simulink model "stabilization"  (R2022b)
settings: Solver=ode14x  StartTime=0.0  StopTime=100  RelTol=1e-3  EnableMultiTasking=on
InitFcn:
  | load regulator.mat
  | load rand_stabilisation.mat
values from neighbouring files (symbols this model uses):
  P = [1 -2 2; -1 2 -1; 1 1 0]    [rand_stabilisation.m]
  Q = transpose([0 0 1])    [rand_stabilisation.m]
undefined symbols (not defined in the file or in its folder): C
settings Model: Creator=torre  LastModifiedBy=anver
settings SolverCC: AlgebraicLoopSolver=TrustRegion  AutoInsertRateTranBlk=on
settings DataIOCC: SaveOutput=off  SaveTime=off
settings OptimizationCC: DefaultParameterBehavior=Inlined  InlineInvariantSignals=on  EnhancedBackFolding=on  PassReuseOutputArgsAs=Individual arguments  StateBitsets=on  DataBitsets=on  ZeroExternalMemoryAtStartup=off  ZeroInternalMemoryAtStartup=off  NoFixptDivByZeroProtection=on  LifeSpan=1  OptimizeBlockOrder=speed  DifferentSizesBufferReuse=on  EfficientTunableParamExpr=on
settings DebuggingCC: ParameterTunabilityLossMsg=error  UnconnectedInputMsg=warning  UnconnectedOutputMsg=warning  UnconnectedLineMsg=warning
settings HardwareCC: ProdBitPerPointer=32  ProdBitPerSizeT=32  ProdBitPerPtrDiffT=32  ProdLargestAtomicFloat=None  ProdIntDivRoundTo=Floor  ProdWordSize=32  ProdHWDeviceType=Generic->Custom
settings ModelReferenceCC: EnableRefExpFcnMdlSchedulingChecks=on
settings SFSimCC: MATLABDynamicMemAlloc=off
settings RTWCC: Description=Embedded Coder  SystemTargetFile=ert.tlc  TLCOptions=-p0  GenCodeOnly=on  TemplateMakefile=ert_default_tmf  GenerateReport=on  RTWVerbose=off  IncludeHyperlinkInReport=on  LaunchReport=on  DLArmComputeVersion=19.05
settings CodeAppCC: ForceParamTrailComments=on  IgnoreCustomStorageClasses=off  OperatorAnnotations=on  SimulinkDataObjDesc=on  SFDataObjDesc=on  CustomSymbolStrGlobalVar=rt$N$M  CustomSymbolStrType=$N$M  CustomSymbolStrFcn=$N$M$F  CustomSymbolStrMacro=$N$M  InsertBlockDesc=on
settings ERTTargetCC: TargetLangStandard=C99 (ISO)  CodeReplacementLibrary=ISO_C  GenerateSampleERTMain=on  IncludeMdlTerminateFcn=off  SuppressErrorStatus=on  SupportAbsoluteTime=off  PurelyIntegerCode=on  SupportNonFinite=off  SupportComplex=off  InlinedParameterPlacement=NonHierarchical  RootIOFormat=Structure reference  ERTCustomFileTemplate=example_file_process.tlc

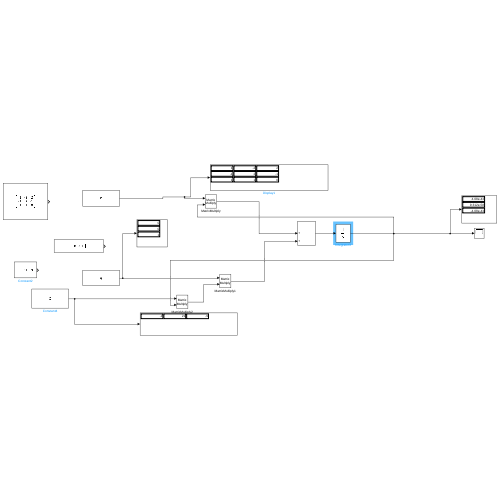
[thumbnail: Simulink's stored preview of the top-level diagram]
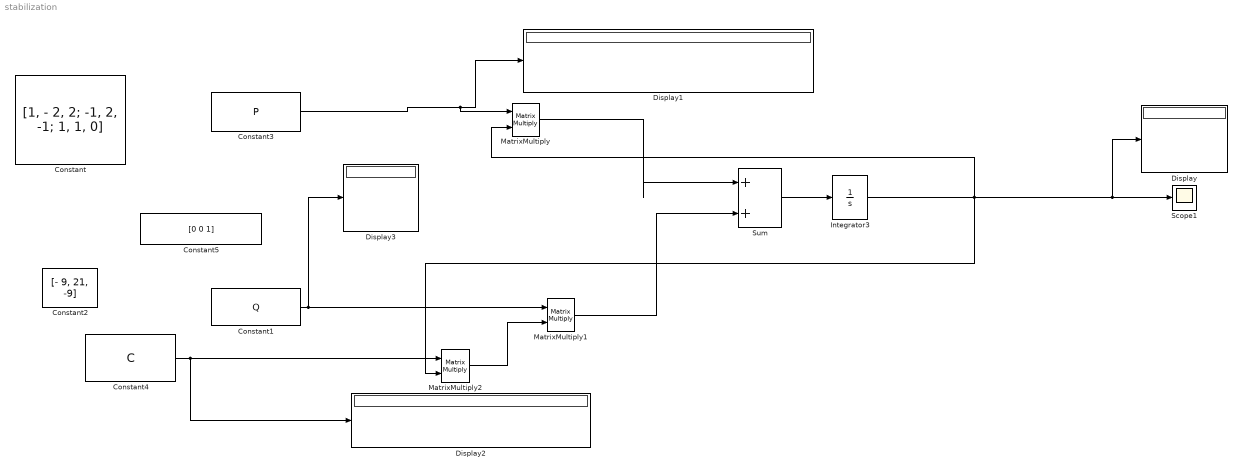
== system stabilization ==
  Constant : Constant  Value="[1, - 2, 2; -1, 2, -1;  1, 1, 0]"  VectorParams1D=off
  Constant1 : Constant  Value=Q  VectorParams1D=off
  Constant2 : Constant  Value=[- 9, 21, -9]
  Constant3 : Constant  Value=P  VectorParams1D=off
  Constant4 : Constant  Value=C  VectorParams1D=off
  Constant5 : Constant  Value=[0 0 1]
  Display{,1..3} (4 alike) : Display
  Integrator3 : Integrator  InitialCondition=1
  MatrixMultiply : Product  Multiplication=Matrix(*)
  MatrixMultiply1 : Product  Multiplication=Matrix(*)
  MatrixMultiply2 : Product  Multiplication=Matrix(*)
  Scope1 : Scope
  Sum : Sum  Inputs=|++
  wires:
  Integrator3/1 -> MatrixMultiply2/2, MatrixMultiply/2, Display/1, Scope1/1
  MatrixMultiply1/1 -> Sum/2
  Sum/1 -> Integrator3/1
  MatrixMultiply/1 -> Sum/1
  MatrixMultiply2/1 -> MatrixMultiply1/2
  Constant3/1 -> MatrixMultiply/1, Display1/1
  Constant1/1 -> Display3/1, MatrixMultiply1/1
  Constant4/1 -> Display2/1, MatrixMultiply2/1
